simulink model "day10p2"  (R2026a)
settings: Solver=FixedStepDiscrete  StopTime=inf
InitFcn:
  | % lmpCntMax = 6;
  | lmpCntMax = 10;
  | % btnCntMax = 10;
  | btnCntMax = 16;
  | % btnStrMax = 39;
  | btnStrMax = 181;
  | % jltStrMax = 17;
  | jltStrMax = 39;
  | lmpStrMax = lmpCntMax + 2;
  | possibilities = dec2bin([0:((2^btnCntMax) - 1)]) - '0';
  | [~, ixs] = sort(sum(possibilities, 2));
  | possibilities = possibilities(ixs, :);
undefined symbols (not defined in the file): DiscIntNeverNeededParam
libraries: simulink x12
(part 2 of 2)

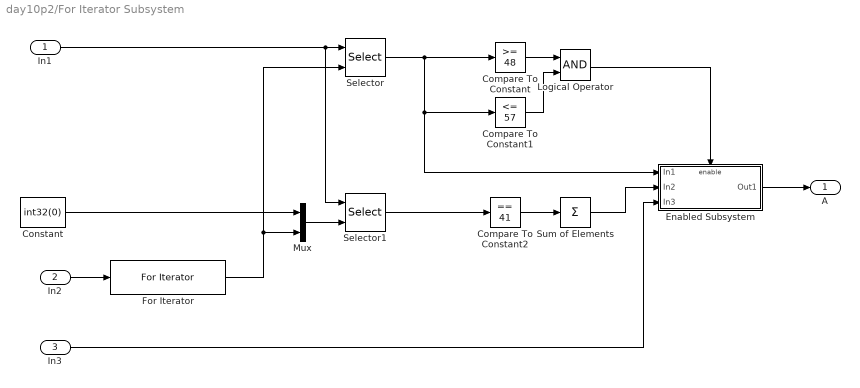
== system day10p2/For Iterator Subsystem ==
  In1 : Inport
  In2 : Inport  Port=2
  In3 : Inport  Port=3
  Compare To Constant : simulink/Logic and Bit Operations/Compare To Constant  relop=>=  const=48  OutDataTypeStr=boolean
  Compare To Constant1 : simulink/Logic and Bit Operations/Compare To Constant  relop=<=  const=57  OutDataTypeStr=boolean
  Compare To Constant2 : simulink/Logic and Bit Operations/Compare To Constant  relop===  const=41  OutDataTypeStr=boolean
  Constant : Constant  Value=int32(0)
  Enabled Subsystem : Subsystem  TreatAsAtomicUnit=on
  For Iterator : ForIterator  ResetStates=reset  IterationSource=external  IndexMode=Zero-based
  Logical Operator : Logic  AllPortsSameDT=off  OutDataTypeStr=boolean
  Mux : Mux  Inputs=2
  Selector : Selector  IndexMode=Zero-based  InputPortWidth=btnStrMax  IndexOptions=Index vector (port)  Indices=[1 3]  OutputSizes=1  RuntimeRangeChecks=on
  Selector1 : Selector  IndexMode=Zero-based  InputPortWidth=btnStrMax  IndexOptions=Starting and ending indices (port)  Indices=[1 3]  OutputSizes=1  RuntimeRangeChecks=on
  Sum of Elements : Sum  Inputs=+
  A : Outport
  wires:
  In2/1 -> For Iterator/1
  Constant/1 -> Mux/1
  For Iterator/1 -> Selector/2, Mux/2
  In1/1 -> Selector1/1, Selector/1
  Mux/1 -> Selector1/2
  Selector/1 -> Enabled Subsystem/1(In1), Compare To Constant1/1, Compare To Constant/1
  Compare To Constant/1 -> Logical Operator/1
  Compare To Constant1/1 -> Logical Operator/2
  Selector1/1 -> Compare To Constant2/1
  Compare To Constant2/1 -> Sum of Elements/1
  Logical Operator/1 -> Enabled Subsystem/Enable
  Enabled Subsystem/1(Out1) -> A/1
  Sum of Elements/1 -> Enabled Subsystem/2(In2)
  In3/1 -> Enabled Subsystem/3(In3)

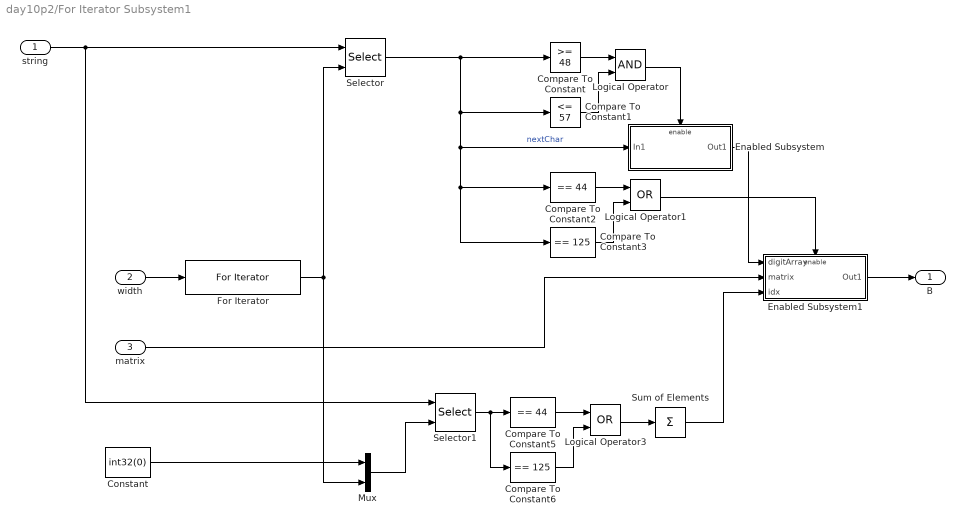
== system day10p2/For Iterator Subsystem1 ==
  string : Inport
  width : Inport  Port=2
  matrix : Inport  Port=3
  Compare To Constant : simulink/Logic and Bit Operations/Compare To Constant  relop=>=  const=48  OutDataTypeStr=boolean
  Compare To Constant1 : simulink/Logic and Bit Operations/Compare To Constant  relop=<=  const=57  OutDataTypeStr=boolean
  Compare To Constant2 : simulink/Logic and Bit Operations/Compare To Constant  relop===  const=44  OutDataTypeStr=boolean
  Compare To Constant3 : simulink/Logic and Bit Operations/Compare To Constant  relop===  const=125  OutDataTypeStr=boolean
  Compare To Constant5 : simulink/Logic and Bit Operations/Compare To Constant  relop===  const=44  OutDataTypeStr=boolean
  Compare To Constant6 : simulink/Logic and Bit Operations/Compare To Constant  relop===  const=125  OutDataTypeStr=boolean
  Constant : Constant  Value=int32(0)
  Enabled Subsystem : Subsystem  TreatAsAtomicUnit=on
  Enabled Subsystem1 : Subsystem  TreatAsAtomicUnit=on
  For Iterator : ForIterator  ResetStates=reset  IterationSource=external  IndexMode=Zero-based
  Logical Operator : Logic  AllPortsSameDT=off  OutDataTypeStr=boolean
  Logical Operator1 : Logic  Operator=OR  AllPortsSameDT=off  OutDataTypeStr=boolean
  Logical Operator3 : Logic  Operator=OR  AllPortsSameDT=off  OutDataTypeStr=boolean
  Mux : Mux  Inputs=2
  Selector : Selector  IndexMode=Zero-based  InputPortWidth=jltStrMax  IndexOptions=Index vector (port)  Indices=[1 3]  OutputSizes=1  RuntimeRangeChecks=on
  Selector1 : Selector  IndexMode=Zero-based  InputPortWidth=jltStrMax  IndexOptions=Starting and ending indices (port)  Indices=[1 3]  OutputSizes=1  RuntimeRangeChecks=on
  Sum of Elements : Sum  Inputs=+
  B : Outport
  wires:
  width/1 -> For Iterator/1
  string/1 -> Selector1/1, Selector/1
  For Iterator/1 -> Selector/2, Mux/2
  Selector/1 -> Compare To Constant3/1, Compare To Constant2/1, Enabled Subsystem/1(In1), Compare To Constant1/1, Compare To Constant/1  "nextChar"
  Compare To Constant/1 -> Logical Operator/1
  Compare To Constant1/1 -> Logical Operator/2
  Logical Operator/1 -> Enabled Subsystem/Enable
  Compare To Constant3/1 -> Logical Operator1/2
  Compare To Constant2/1 -> Logical Operator1/1
  Logical Operator1/1 -> Enabled Subsystem1/Enable
  Enabled Subsystem/1(Out1) -> Enabled Subsystem1/1(digitArray)
  Enabled Subsystem1/1(Out1) -> B/1
  matrix/1 -> Enabled Subsystem1/2(matrix)
  Mux/1 -> Selector1/2
  Constant/1 -> Mux/1
  Sum of Elements/1 -> Enabled Subsystem1/3(idx)
  Compare To Constant5/1 -> Logical Operator3/1
  Compare To Constant6/1 -> Logical Operator3/2
  Selector1/1 -> Compare To Constant6/1, Compare To Constant5/1
  Logical Operator3/1 -> Sum of Elements/1

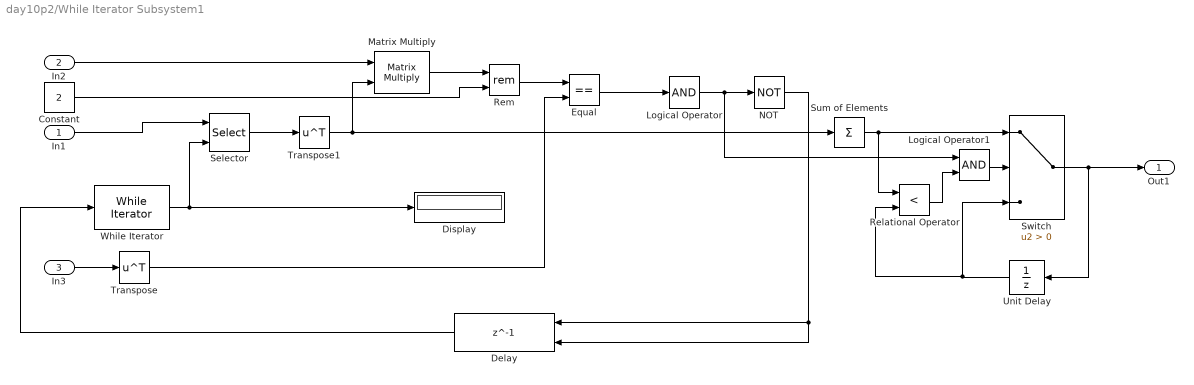
== system day10p2/While Iterator Subsystem1 ==
  In1 : Inport
  In2 : Inport  Port=2
  In3 : Inport  Port=3
  Constant : Constant  Value=2
  Delay : Delay  DelayLength=1  InitialConditionSource=Input port
      settings: InputPortMap=u0,p4
  Display : Display
  Equal : RelationalOperator  Operator===  OutDataTypeStr=boolean  RndMeth=Simplest  InputSameDT=off
  Logical Operator : Logic  Inputs=1  AllPortsSameDT=off  OutDataTypeStr=boolean
  Logical Operator1 : Logic  AllPortsSameDT=off  OutDataTypeStr=boolean
  Matrix Multiply : Product  Multiplication=Matrix(*)
  NOT : Logic  Operator=NOT  IconShape=distinctive  AllPortsSameDT=off  OutDataTypeStr=boolean
  Relational Operator : RelationalOperator  Operator=<  OutDataTypeStr=boolean  RndMeth=Simplest  InputSameDT=off
  Rem : Math  Operator=rem
  Selector : Selector  NumberOfDimensions=2  InputPortWidth=3  IndexOptions=Index vector (port),Select all  Indices=[1 3],1  OutputSizes=1,1  RuntimeRangeChecks=on
  Sum of Elements : Sum  Inputs=+
  Switch : Switch  Criteria=u2 > Threshold  SaturateOnIntegerOverflow=off  InputSameDT=off
  Transpose : Math  Operator=transpose
  Transpose1 : Math  Operator=transpose
  Unit Delay : UnitDelay  InitialCondition=Inf  SampleTime=-1
  While Iterator : WhileIterator  MaxIters=-1  WhileBlockType=do-while  ResetStates=reset  ShowIterationPort=on
  Out1 : Outport
  wires:
  In3/1 -> Transpose/1
  In1/1 -> Selector/1
  While Iterator/1 -> Display/1, Selector/2
  Selector/1 -> Transpose1/1
  In2/1 -> Matrix Multiply/1
  Transpose1/1 -> Sum of Elements/1, Matrix Multiply/2
  Matrix Multiply/1 -> Rem/1
  Constant/1 -> Rem/2
  Rem/1 -> Equal/1
  Transpose/1 -> Equal/2
  Equal/1 -> Logical Operator/1
  Logical Operator/1 -> Logical Operator1/1, NOT/1
  NOT/1 -> Delay/2, Delay/1
  Delay/1 -> While Iterator/1
  Switch/1 -> Out1/1, Unit Delay/1
  Sum of Elements/1 -> Relational Operator/1, Switch/1
  Logical Operator1/1 -> Switch/2
  Relational Operator/1 -> Logical Operator1/2
  Unit Delay/1 -> Switch/3, Relational Operator/2

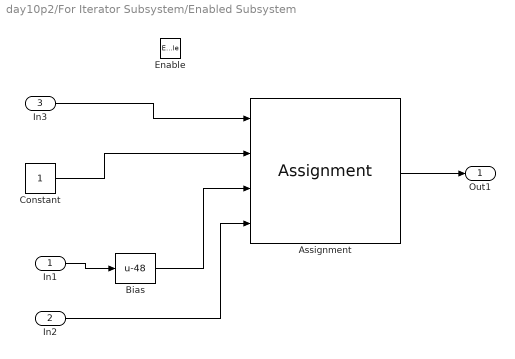
== system day10p2/For Iterator Subsystem/Enabled Subsystem ==
  In1 : Inport
  In2 : Inport  Port=2
  In3 : Inport  Port=3
  Enable : EnablePort  StatesWhenEnabling=reset
  Assignment : Assignment  NumberOfDimensions=2  IndexMode=Zero-based  DiagnosticForDimensions=Warning  IndexOptions=Index vector (port),Index vector (port)  Indices=1,1  OutputSizes=1,1  RuntimeRangeChecks=on
  Bias : Bias  Bias=-48  SaturateOnIntegerOverflow=off
  Constant : Constant
  Out1 : Outport
  wires:
  In1/1 -> Bias/1
  In3/1 -> Assignment/1
  Constant/1 -> Assignment/2
  Bias/1 -> Assignment/3
  In2/1 -> Assignment/4
  Assignment/1 -> Out1/1

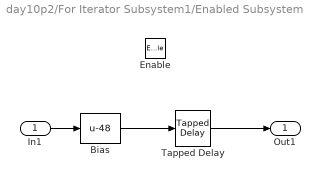
== system day10p2/For Iterator Subsystem1/Enabled Subsystem ==
  In1 : Inport
  Enable : EnablePort  StatesWhenEnabling=reset
  Bias : Bias  Bias=-48  SaturateOnIntegerOverflow=off
  Tapped Delay : simulink/Discrete/Tapped Delay  vinit=0.0  samptime=-1  NumDelays=3  DelayOrder=Oldest  includeCurrent=on
  Out1 : Outport
  wires:
  In1/1 -> Bias/1
  Tapped Delay/1 -> Out1/1
  Bias/1 -> Tapped Delay/1

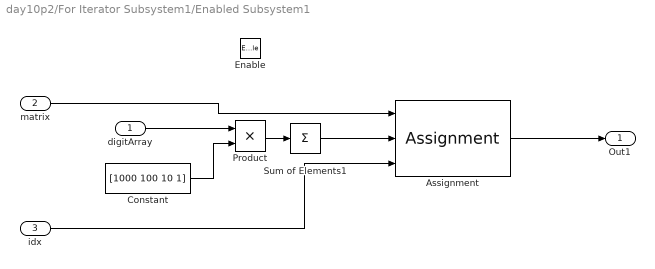
== system day10p2/For Iterator Subsystem1/Enabled Subsystem1 ==
  digitArray : Inport
  matrix : Inport  Port=2
  idx : Inport  Port=3
  Enable : EnablePort  StatesWhenEnabling=reset
  Assignment : Assignment  DiagnosticForDimensions=Warning  IndexOptions=Index vector (port)  Indices=1  OutputSizes=1  RuntimeRangeChecks=on
  Constant : Constant  Value=[1000 100 10 1]
  Product : Product
  Sum of Elements1 : Sum  Inputs=+
  Out1 : Outport
  wires:
  digitArray/1 -> Product/1
  Constant/1 -> Product/2
  Product/1 -> Sum of Elements1/1
  matrix/1 -> Assignment/1
  Assignment/1 -> Out1/1
  Sum of Elements1/1 -> Assignment/2
  idx/1 -> Assignment/3

== matlab function day10p2/MATLAB Function ==
  data: A input; X output; B input
function X = fcn(A, B)

X = linsolve(A, B);
